simulink subsystem "LinezInZero"  (R2023a)
settings: Solver=VariableStepAuto  StartTime=0.0  StopTime=10.0  RelTol=1e-3
settings Model: Creator=ycheb  LastModifiedBy=ycheb

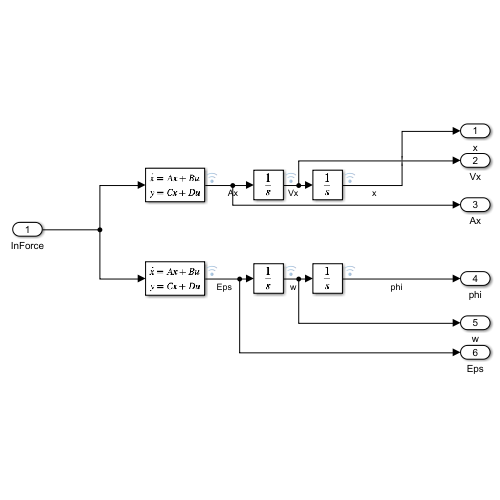
[thumbnail: Simulink's stored preview of the top-level diagram]
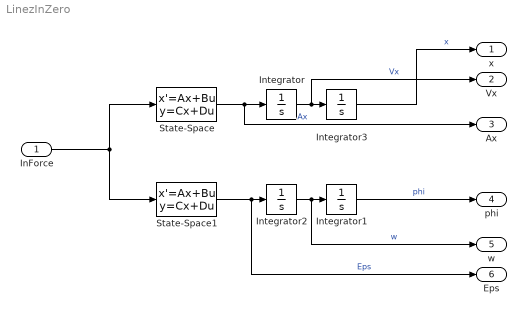
== system LinezInZero ==
  InForce : Inport
  Integrator : Integrator
  Integrator1 : Integrator  InitialCondition=-5*pi/180
  Integrator2 : Integrator
  Integrator3 : Integrator
  State-Space : StateSpace  A=[1,0,0,-0.00326666666661222;0.001,1,0,-1.63333333330611e-06;0,0,1,0.0098;0,0,0.001,1]  B=[0.004444444444444;2.222222222222221e-06;-0.003333337416668;-1.666667687500250e-06]  C=[0,0,0,-3.266666666612221]  D=4.444444444444442  InitialCondition=0
  State-Space1 : StateSpace  A=[1,0,0,-0.00326666666661222;0.00100000000000000,1,0,-1.63333333330611e-06;0,0,1,0.0098;0,0,0.001,1]  B=[0.004444444444444;2.222222222222221e-06;-0.003333337416668;-1.666667687500250e-06]  C=[0,0,0,9.799999999836665]  D=-3.333333333333332  InitialCondition=0
  x : Outport
  Vx : Outport  Port=2
  Ax : Outport  Port=3
  phi : Outport  Port=4
  w : Outport  Port=5
  Eps : Outport  Port=6
  wires:
  Integrator3/1 -> x/1  "x"
  Integrator/1 -> Integrator3/1, Vx/1  "Vx"
  State-Space/1 -> Integrator/1, Ax/1  "Ax"
  Integrator2/1 -> Integrator1/1, w/1  "w"
  Integrator1/1 -> phi/1  "phi"
  State-Space1/1 -> Integrator2/1, Eps/1  "Eps"
  InForce/1 -> State-Space/1, State-Space1/1
